simulink model "TVModel_Simulation_21"  (R2021b)
settings: Solver=FixedStepDiscrete  StartTime=0.0  StopTime=250  FixedStep=0.02  MaxStep=0.01  RelTol=1e-3
undefined symbols (not defined in the file or in its folder): MB, TV, TV_OLD
libraries: simulink x22, simulink_extras x14, eeGeneralControl x13, slpidlib x8, fuzblock x4, controlLib x4, cstblocks x3, dspstat3 x2, eeSlidingModeController x1, sharedTrackingLibrary x1
(part 2 of 9)

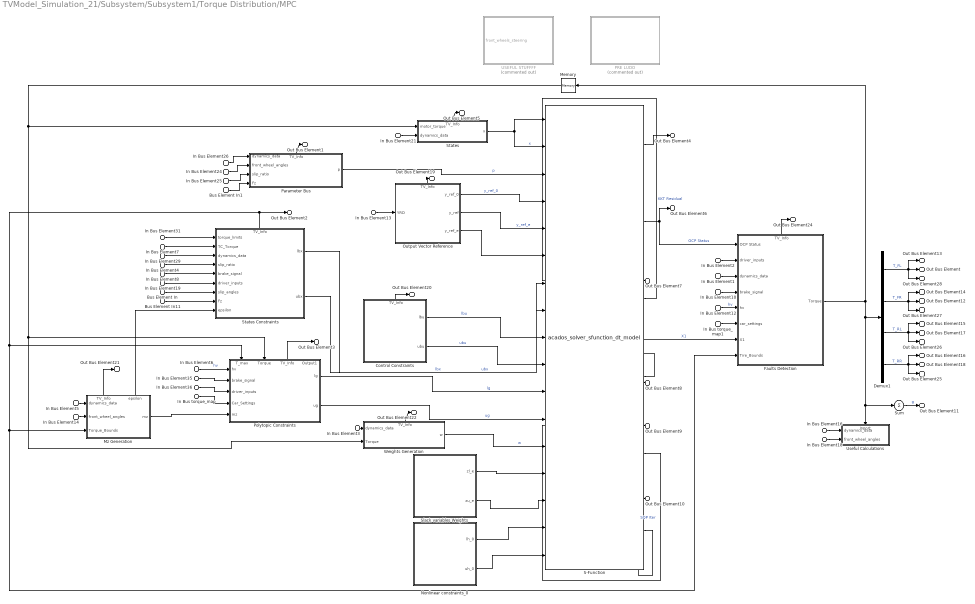
== system TVModel_Simulation_21/Subsystem/Subsystem1/Torque Distribution/MPC ==
  In Bus Element31 : Inport  PortName=torque_limits
  In Bus Element{1,3,5,16,21,26,29} (7 alike) : Inport  Port=2  PortName=dynamics_data
  In Bus Element13 : Inport  Port=3  PortName=yaw_rate_desired
  In Bus Element25 : Inport  Port=4  PortName=slip_ratio
  In Bus Element4 : Inport  Port=4  PortName=slip_ratio
  In Bus Element36 : Inport  Port=5  PortName=driver_inputs
  In Bus Element2 : Inport  Port=5  PortName=driver_inputs
  In Bus Element19 : Inport  Port=5  PortName=driver_inputs
  In Bus Element24 : Inport  Port=6  PortName=front_wheel_angles
  In Bus Element14 : Inport  Port=6  PortName=front_wheel_angles
  In Bus Element18 : Inport  Port=6  PortName=front_wheel_angles
  In Bus Element35 : Inport  Port=7  PortName=brake_signal
  In Bus Element8 : Inport  Port=7  PortName=brake_signal
  In Bus Element10 : Inport  Port=7  PortName=brake_signal
  In Bus Element7 : Inport  Port=8  PortName=TC_Torque
  In Bus torque_map : Inport  Port=9  PortName=Car_Setting
  In Bus torque_map1 : Inport  Port=9  PortName=Car_Setting
  In Bus Element6 : Inport  Port=10  PortName=hv
  In Bus Element12 : Inport  Port=10  PortName=hv
  Bus Element In : Inport  Port=11  PortName=slip_angles
  Bus Element In11 : Inport  Port=12  PortName=Fz
  Bus Element In1 : Inport  Port=12  PortName=Fz
  "     Output Vector Reference" : Subsystem
      settings: PortSchema="{\"entries\":[{\"content\":{\"sides\":[{\"content\":{\"connectorIds\":[\"In1\"]},\"type\":\"ConnectorPlacement.EquallySpacedRectSide\",\"uuid\":\"6eb43855-e5bb-45e2-8cd4-f053b217ea66\"},{\"content\":{\"connectorIds\":[\"Out1\",\"Out2\",\"Out3\"],\"side\":\"RIGHT\"},\"type\":\"ConnectorPlacement.EquallySpacedRectSide\",\"uuid\":\"38094b7e-63b6-42ff-9f99-20977d79efed\"},{\"content\":{\"connectorIds\":[\"Out4\"],\"side\":\"TOP\"},\"type\":\"ConnectorPlacement.EquallySpacedRectSide\",\"uuid\":\"9a3bf522-481b-4973-827b-befc16d2412c\"}]},\"type\":\"ConnectorPlacement.EquallySpacedConnector\",\"uuid\":\"c4e1068e-763d-4b01-8680-18fb7e18710b\"}],\"packageUris\":[\"http://schema.mathworks.com/mf0/Connector/R2020b\"],\"version\":\"1.0\"}"
  " PRE LUDO" : Subsystem  Commented=on
  " Parameter Bus " : Subsystem
      settings: PortSchema="{\"entries\":[{\"content\":{\"sides\":[{\"content\":{\"connectorIds\":[\"In1\",\"In2\",\"In3\",\"In4\"]},\"type\":\"ConnectorPlacement.EquallySpacedRectSide\",\"uuid\":\"a09562f1-0ace-4da8-b0ba-541877c845d4\"},{\"content\":{\"connectorIds\":[\"Out1\"],\"side\":\"RIGHT\"},\"type\":\"ConnectorPlacement.EquallySpacedRectSide\",\"uuid\":\"f2ac5cc5-a3cf-4f44-b665-78a7b5313457\"},{\"content\":{\"connectorIds\":[\"Out2\"],\"side\":\"TOP\"},\"type\":\"ConnectorPlacement.EquallySpacedRectSide\",\"uuid\":\"e9b1b537-1334-4243-8de4-5033dcf158b3\"}]},\"type\":\"ConnectorPlacement.EquallySpacedConnector\",\"uuid\":\"4a13e9e0-d022-4af6-9a72-5499c727e49d\"}],\"packageUris\":[\"http://schema.mathworks.com/mf0/Connector/R2020b\"],\"version\":\"1.0\"}"
  " States" : Subsystem
      settings: PortSchema="{\"entries\":[{\"content\":{\"sides\":[{\"content\":{\"connectorIds\":[\"In1\",\"In2\"]},\"type\":\"ConnectorPlacement.EquallySpacedRectSide\",\"uuid\":\"8d332d78-bc9f-4997-8663-87f4f2365fc7\"},{\"content\":{\"connectorIds\":[\"Out1\"],\"side\":\"RIGHT\"},\"type\":\"ConnectorPlacement.EquallySpacedRectSide\",\"uuid\":\"d5a2d93d-05d2-4fab-b578-55a6b40e1b7e\"},{\"content\":{\"connectorIds\":[\"Out2\"],\"side\":\"TOP\"},\"type\":\"ConnectorPlacement.EquallySpacedRectSide\",\"uuid\":\"85119e7a-0f7b-42a4-aa47-c419ac915ed1\"}]},\"type\":\"ConnectorPlacement.EquallySpacedConnector\",\"uuid\":\"bc00bdd8-907b-4556-9b65-7ae115265b2a\"}],\"packageUris\":[\"http://schema.mathworks.com/mf0/Connector/R2020b\"],\"version\":\"1.0\"}"
  Control Constraints : Subsystem
      settings: PortSchema="{\"entries\":[{\"content\":{\"sides\":[{\"content\":{\"connectorIds\":[]},\"type\":\"ConnectorPlacement.EquallySpacedRectSide\",\"uuid\":\"3047f7f6-6911-4b59-830a-220636e586ba\"},{\"content\":{\"connectorIds\":[\"Out1\",\"Out2\"],\"side\":\"RIGHT\"},\"type\":\"ConnectorPlacement.EquallySpacedRectSide\",\"uuid\":\"8d090d6d-9b64-48c1-acb0-b5c53a8577b5\"},{\"content\":{\"connectorIds\":[\"Out3\"],\"side\":\"TOP\"},\"type\":\"ConnectorPlacement.EquallySpacedRectSide\",\"uuid\":\"2db0e490-1b70-46d0-9c30-5c7bdf8b2a28\"}]},\"type\":\"ConnectorPlacement.EquallySpacedConnector\",\"uuid\":\"45990a81-75f2-4fb4-b041-5594cb9ed930\"}],\"packageUris\":[\"http://schema.mathworks.com/mf0/Connector/R2020b\"],\"version\":\"1.0\"}"
  Demux1 : Demux
  Faults Detection : Subsystem
      settings: PortSchema="{\"entries\":[{\"content\":{\"sides\":[{\"content\":{\"connectorIds\":[\"In1\",\"In2\",\"In3\",\"In4\",\"In5\",\"In6\",\"In7\",\"In8\"]},\"type\":\"ConnectorPlacement.EquallySpacedRectSide\",\"uuid\":\"334783ee-11f3-4144-8a14-28dc56086a4b\"},{\"content\":{\"connectorIds\":[\"Out1\"],\"side\":\"RIGHT\"},\"type\":\"ConnectorPlacement.EquallySpacedRectSide\",\"uuid\":\"49c8e620-bd09-4fee-a8d6-6c7a5f6563c1\"},{\"content\":{\"connectorIds\":[\"Out2\"],\"side\":\"TOP\"},\"type\":\"ConnectorPlacement.EquallySpacedRectSide\",\"uuid\":\"cef52ef8-f6f7-4321-a9c9-502de0ffc851\"}]},\"type\":\"ConnectorPlacement.EquallySpacedConnector\",\"uuid\":\"45428ca6-b9a3-4f64-8f7b-2072997d615d\"}],\"packageUris\":[\"http://schema.mathworks.com/mf0/Connector/R2020b\"],\"version\":\"1.0\"}"
  Memory : Memory  InheritSampleTime=on
  Mz Generation : Subsystem
      settings: PortSchema="{\"entries\":[{\"content\":{\"sides\":[{\"content\":{\"connectorIds\":[\"In1\",\"In2\",\"In3\"]},\"type\":\"ConnectorPlacement.EquallySpacedRectSide\",\"uuid\":\"12822615-03ad-45f6-8c43-45acae00b3c9\"},{\"content\":{\"connectorIds\":[\"Out1\"],\"side\":\"RIGHT\"},\"type\":\"ConnectorPlacement.EquallySpacedRectSide\",\"uuid\":\"651d1d31-9a4c-422b-aacb-e7edf3ade298\"},{\"content\":{\"connectorIds\":[\"Out2\",\"Out3\"],\"side\":\"TOP\"},\"type\":\"ConnectorPlacement.EquallySpacedRectSide\",\"uuid\":\"d0f71465-89ce-4a1f-947c-d935b63c1581\"}]},\"type\":\"ConnectorPlacement.EquallySpacedConnector\",\"uuid\":\"d07c68d3-c928-4ca4-a746-c386ba32e252\"}],\"packageUris\":[\"http://schema.mathworks.com/mf0/Connector/R2020b\"],\"version\":\"1.0\"}"
  Nonlinear constraints_0 : Subsystem
  Polytopic Constraints : Subsystem
      settings: PortSchema="{\"entries\":[{\"content\":{\"sides\":[{\"content\":{\"connectorIds\":[\"In1\",\"In2\",\"In3\",\"In4\",\"In5\"]},\"type\":\"ConnectorPlacement.EquallySpacedRectSide\",\"uuid\":\"e13c359e-3a3f-4544-8ddb-27eff3db9dcd\"},{\"content\":{\"connectorIds\":[\"Out1\",\"Out2\"],\"side\":\"RIGHT\"},\"type\":\"ConnectorPlacement.EquallySpacedRectSide\",\"uuid\":\"2a9e23e2-ef2f-461f-adc6-9f7488968d10\"},{\"content\":{\"connectorIds\":[\"In6\",\"In7\",\"Out3\",\"Out4\"],\"side\":\"TOP\"},\"type\":\"ConnectorPlacement.EquallySpacedRectSide\",\"uuid\":\"7b13a6d7-9b26-4287-8cf5-02c8da23c4d1\"}]},\"type\":\"ConnectorPlacement.EquallySpacedConnector\",\"uuid\":\"8c73910d-15b7-446d-b267-8db7451f6e4d\"}],\"packageUris\":[\"http://schema.mathworks.com/mf0/Connector/R2020b\"],\"version\":\"1.0\"}"
  S-Function : S-Function  FunctionName=acados_solver_sfunction_dt_model  SFunctionDeploymentMode=off  EnableBusSupport=off
  "Slack variables Weights " : Subsystem
  States Constraints : Subsystem
      settings: PortSchema="{\"entries\":[{\"content\":{\"sides\":[{\"content\":{\"connectorIds\":[\"In1\",\"In2\",\"In3\",\"In4\",\"In5\",\"In6\",\"In7\",\"In8\",\"In9\"]},\"type\":\"ConnectorPlacement.EquallySpacedRectSide\",\"uuid\":\"79113e7a-8644-4397-b81a-3f4227f55e88\"},{\"content\":{\"connectorIds\":[\"Out1\",\"Out2\"],\"side\":\"RIGHT\"},\"type\":\"ConnectorPlacement.EquallySpacedRectSide\",\"uuid\":\"08be16f7-b5e6-4d72-833b-a0e4a6b6f372\"},{\"content\":{\"connectorIds\":[\"Out3\"],\"side\":\"TOP\"},\"type\":\"ConnectorPlacement.EquallySpacedRectSide\",\"uuid\":\"49b46e5c-f00c-463e-b91e-3df34e18eb9d\"}]},\"type\":\"ConnectorPlacement.EquallySpacedConnector\",\"uuid\":\"b55b5f62-a08b-4632-a68f-4c31f9c7626d\"}],\"packageUris\":[\"http://schema.mathworks.com/mf0/Connector/R2020b\"],\"version\":\"1.0\"}"
  Sum : Sum  Inputs=+
  USEFUL STUFFFF : Subsystem  Commented=on
  Useful Calculations : Subsystem
      settings: PortSchema="{\"entries\":[{\"content\":{\"sides\":[{\"content\":{\"connectorIds\":[\"In1\",\"In2\"]},\"type\":\"ConnectorPlacement.EquallySpacedRectSide\",\"uuid\":\"a16c8cbd-7e59-4ceb-ae2f-8328deb35aba\"},{\"content\":{\"connectorIds\":[],\"side\":\"RIGHT\"},\"type\":\"ConnectorPlacement.EquallySpacedRectSide\",\"uuid\":\"ab644b37-73a3-4dcd-8f59-2df4491a3297\"},{\"content\":{\"connectorIds\":[\"In3\"],\"side\":\"TOP\"},\"type\":\"ConnectorPlacement.EquallySpacedRectSide\",\"uuid\":\"9843ece7-aa20-4f32-a700-0380b8b7d47e\"}]},\"type\":\"ConnectorPlacement.EquallySpacedConnector\",\"uuid\":\"e857cd10-f7b6-4e82-8686-4c399562f8ce\"}],\"packageUris\":[\"http://schema.mathworks.com/mf0/Connector/R2020b\"],\"version\":\"1.0\"}"
  Weights Generation : Subsystem
      settings: PortSchema="{\"entries\":[{\"content\":{\"sides\":[{\"content\":{\"connectorIds\":[\"In1\",\"In2\"]},\"type\":\"ConnectorPlacement.EquallySpacedRectSide\",\"uuid\":\"334783ee-11f3-4144-8a14-28dc56086a4b\"},{\"content\":{\"connectorIds\":[\"Out1\"],\"side\":\"RIGHT\"},\"type\":\"ConnectorPlacement.EquallySpacedRectSide\",\"uuid\":\"49c8e620-bd09-4fee-a8d6-6c7a5f6563c1\"},{\"content\":{\"connectorIds\":[\"Out2\"],\"side\":\"TOP\"},\"type\":\"ConnectorPlacement.EquallySpacedRectSide\",\"uuid\":\"cef52ef8-f6f7-4321-a9c9-502de0ffc851\"}]},\"type\":\"ConnectorPlacement.EquallySpacedConnector\",\"uuid\":\"45428ca6-b9a3-4f64-8f7b-2072997d615d\"}],\"packageUris\":[\"http://schema.mathworks.com/mf0/Connector/R2020b\"],\"version\":\"1.0\"}"
  Out Bus Element5 : Outport  PortName=TV_Info  Element=States
  Out Bus Element2 : Outport  PortName=TV_Info  Element=States_Constraints
  Out Bus Element3 : Outport  PortName=TV_Info  Element=Polytopic Constraints
  Out Bus Element4 : Outport  PortName=TV_Info  Element=control
  Out Bus Element6 : Outport  PortName=TV_Info  Element=Solver.OCP_status
  Out Bus Element7 : Outport  PortName=TV_Info  Element=Solver.KKT_Residual
  Out Bus Element8 : Outport  PortName=TV_Info  Element=Solver.X1
  Out Bus Element9 : Outport  PortName=TV_Info  Element=Solver.CPU_time
  Out Bus Element10 : Outport  PortName=TV_Info  Element=Solver.SQP_iter
  Out Bus Element16 : Outport  PortName=TV_Info  Element=Torque.t_rr
  Out Bus Element15 : Outport  PortName=TV_Info  Element=Torque.t_rl
  Out Bus Element14 : Outport  PortName=TV_Info  Element=Torque.t_fr
  Out Bus Element13 : Outport  PortName=TV_Info  Element=Torque.t_fl
  Out Bus Element11 : Outport  PortName=TV_Info  Element=Faults.g
  Out Bus Element1 : Outport  PortName=TV_Info  Element=Parameters
  Out Bus Element19 : Outport  PortName=TV_Info  Element=Vector_Reference
  Out Bus Element20 : Outport  PortName=TV_Info  Element=Control_Constraints
  Out Bus Element21 : Outport  PortName=TV_Info  Element=Mz_Saturation
  Out Bus Element22 : Outport  PortName=TV_Info  Element=Weights_Generation
  Out Bus Element24 : Outport  PortName=TV_Info  Element=Faults_Detection
  Out Bus Element : Outport  Port=2  PortName=TV  Element=FL
  Out Bus Element12 : Outport  Port=2  PortName=TV  Element=FR
  Out Bus Element17 : Outport  Port=2  PortName=TV  Element=RL
  Out Bus Element18 : Outport  Port=2  PortName=TV  Element=RR
  Out Bus Element25 : Outport  Port=3  PortName=TC_torque_out  Element=RR
  Out Bus Element26 : Outport  Port=3  PortName=TC_torque_out  Element=RL
  Out Bus Element27 : Outport  Port=3  PortName=TC_torque_out  Element=FR
  Out Bus Element28 : Outport  Port=3  PortName=TC_torque_out  Element=FL
  wires:
  Nonlinear constraints_0/2(uh_0) -> S-Function/17
  " States"/1(x) -> S-Function/1, S-Function/2  "x"
  In Bus Element21/1 -> " States"/2(dynamics_data)
  Mz Generation/3(epsilon) -> States Constraints/9(epsilon)
  In Bus Element18/1 -> Useful Calculations/2(front_wheel_angles)
  In Bus Element16/1 -> Useful Calculations/1(dynamics_data)
  Mz Generation/1(mz) -> Polytopic Constraints/5(mz)
  In Bus torque_map/1 -> Polytopic Constraints/4(Car_Settings)
  In Bus Element2/1 -> Faults Detection/2(driver_inputs)
  In Bus Element1/1 -> Faults Detection/3(dynamics_data)
  In Bus Element36/1 -> Polytopic Constraints/3(driver_inputs)
  In Bus Element35/1 -> Polytopic Constraints/2(brake_signal)
  In Bus Element24/1 -> " Parameter Bus "/2(front_wheel_angles)
  In Bus Element26/1 -> " Parameter Bus "/1(dynamics_data)
  In Bus Element25/1 -> " Parameter Bus "/3(slip_ratio)
  In Bus Element13/1 -> "     Output Vector Reference"/1(YRD)
  S-Function/5 -> Out Bus Element9/1
  S-Function/6 -> Out Bus Element10/1  "SQP Iter"
  S-Function/3 -> Out Bus Element7/1  "KKT Residual"
  S-Function/2 -> Faults Detection/1(OCP Status), Out Bus Element6/1  "OCP Status"
  Sum/1 -> Out Bus Element11/1  "g"
  Memory/1 -> " States"/1(motor_torque), Weights Generation/2(Torque), Polytopic Constraints/7(Torque)
  " States"/2(TV_Info) -> Out Bus Element5/1
  States Constraints/3(TV_Info) -> Faults Detection/8(Tire_Bounds), Mz Generation/3(Torque_Bounds), Polytopic Constraints/6(T_max), Out Bus Element2/1
  Polytopic Constraints/3(TV_Info) -> Out Bus Element3/1
  Demux1/1 -> Out Bus Element28/1, Out Bus Element/1, Out Bus Element13/1  "T_FL"
  Demux1/2 -> Out Bus Element27/1, Out Bus Element12/1, Out Bus Element14/1  "T_FR"
  Demux1/3 -> Out Bus Element26/1, Out Bus Element15/1, Out Bus Element17/1  "T_RL"
  Demux1/4 -> Out Bus Element25/1, Out Bus Element18/1, Out Bus Element16/1  "T_RR"
  In Bus Element3/1 -> Weights Generation/1(dynamics_data)
  S-Function/1 -> Out Bus Element4/1
  In Bus Element6/1 -> Polytopic Constraints/1(hv)  "hv"
  Faults Detection/1(Torque) -> Demux1/1, Sum/1, Useful Calculations/3(Inport), Memory/1
  " Parameter Bus "/2(TV_Info) -> Out Bus Element1/1
  "     Output Vector Reference"/4(TV_Info) -> Out Bus Element19/1
  Control Constraints/3(TV_Info) -> Out Bus Element20/1
  In Bus Element5/1 -> Mz Generation/1(dynamics_data)
  Mz Generation/2(TV_Info) -> Out Bus Element21/1
  Weights Generation/2(TV_Info) -> Out Bus Element22/1
  Faults Detection/2(TV_Info) -> Out Bus Element24/1
  In Bus Element14/1 -> Mz Generation/2(front_wheel_angles)
  In Bus Element12/1 -> Faults Detection/5(hv)  "hv"
  In Bus torque_map1/1 -> Faults Detection/6(car_settings)
  In Bus Element10/1 -> Faults Detection/4(brake_signal)
  Bus Element In11/1 -> States Constraints/8(Fz)
  Bus Element In/1 -> States Constraints/7(slip_angles)
  In Bus Element19/1 -> States Constraints/6(driver_inputs)
  In Bus Element8/1 -> States Constraints/5(brake_signal)
  In Bus Element4/1 -> States Constraints/4(slip_ratio)
  In Bus Element29/1 -> States Constraints/3(dynamics_data)
  In Bus Element7/1 -> States Constraints/2(TC_Torque)
  In Bus Element31/1 -> States Constraints/1(torque_limits)
  S-Function/4 -> Faults Detection/7(X1), Out Bus Element8/1  "X1"
  Bus Element In1/1 -> " Parameter Bus "/4(Fz)
  " Parameter Bus "/1(p) -> S-Function/3  "p"
  "     Output Vector Reference"/1(y_ref_0) -> S-Function/4  "y_ref_0"
  "     Output Vector Reference"/2(y_ref) -> S-Function/5  "y_ref_e"
  "     Output Vector Reference"/3(y_ref_e) -> S-Function/6
  States Constraints/1(lbx) -> S-Function/7  "lbx"
  States Constraints/2(ubx) -> S-Function/8  "ubx"
  Control Constraints/1(lbu) -> S-Function/9  "lbu"
  Control Constraints/2(ubu) -> S-Function/10  "ubu"
  Polytopic Constraints/1(lg) -> S-Function/11  "lg"
  Polytopic Constraints/2(ug) -> S-Function/12  "ug"
  Weights Generation/1(w) -> S-Function/13  "w"
  "Slack variables Weights "/1(zl_e) -> S-Function/14
  "Slack variables Weights "/2(zu_e) -> S-Function/15
  Nonlinear constraints_0/1(lh_0) -> S-Function/16

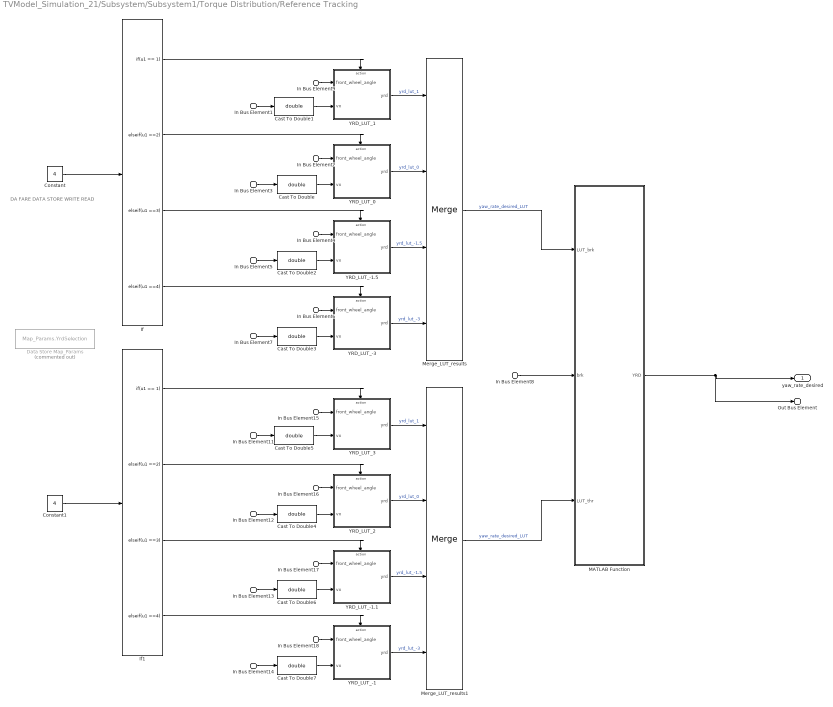
== system TVModel_Simulation_21/Subsystem/Subsystem1/Torque Distribution/Reference Tracking ==
  note: DA FARE DATA STORE WRITE READ
  In Bus Element{1,3,5,7,11..14} (8 alike) : Inport  PortName=dynamics_data  Element=vx
  In Bus Element{2,4,6,9,15..18} (8 alike) : Inport  Port=2  PortName=front_wheels_steering  Element=single_axis
  In Bus Element8 : Inport  Port=3  PortName=driver_inputs  Element=brake
  Cast To Double{,1..7} (8 alike) : DataTypeConversion  OutDataTypeStr=double
  Constant : Constant  Value=4
  Constant1 : Constant  Value=4
  Data Store Map_Params : DataStoreRead  Commented=on  DataStoreName=Map_Params  DataStoreElements=Map_Params.YrdSelection  IndexOptions=Index vector (dialog)  Indices=1  OutputSizes=1
  If : If  IfExpression=u1 == 1  ElseIfExpressions=u1 ==2,u1 ==3,u1 ==4  ShowElse=off
  If1 : If  IfExpression=u1 == 1  ElseIfExpressions=u1 ==2,u1 ==3,u1 ==4  ShowElse=off
  MATLAB Function : MATLAB Function  TreatAsAtomicUnit=on  SystemSampleTime=TV.MPC.T/TV.MPC.N
  Merge_LUT_results : Merge  Inputs=4
  Merge_LUT_results1 : Merge  Inputs=4
  YRD_LUT_-1 : Subsystem  TreatAsAtomicUnit=on
      mask Display: image('Mask_Icon\LUT.png'); % Use "Edit Image" on toolstrip to change.
  YRD_LUT_-1.1 : Subsystem  TreatAsAtomicUnit=on
      mask Display: image('Mask_Icon\LUT.png'); % Use "Edit Image" on toolstrip to change.
  YRD_LUT_-1.5 : Subsystem  TreatAsAtomicUnit=on
      mask Display: image('Mask_Icon\LUT.png'); % Use "Edit Image" on toolstrip to change.
  YRD_LUT_-3 : Subsystem  TreatAsAtomicUnit=on
      mask Display: image('Mask_Icon\LUT.png'); % Use "Edit Image" on toolstrip to change.
  YRD_LUT_0 : Subsystem  TreatAsAtomicUnit=on
      mask Display: image('Mask_Icon\LUT.png'); % Use "Edit Image" on toolstrip to change.
  YRD_LUT_1 : Subsystem  TreatAsAtomicUnit=on
      mask Display: image('Mask_Icon\LUT.png'); % Use "Edit Image" on toolstrip to change.
  YRD_LUT_2 : Subsystem  TreatAsAtomicUnit=on
      mask Display: image('Mask_Icon\LUT.png'); % Use "Edit Image" on toolstrip to change.
  YRD_LUT_3 : Subsystem  TreatAsAtomicUnit=on
      mask Display: image('Mask_Icon\LUT.png'); % Use "Edit Image" on toolstrip to change.
  yaw_rate_desired : Outport
  Out Bus Element : Outport  Port=2  PortName=TV_Info  Element=yaw_rate_desired
  wires:
  MATLAB Function/1(YRD) -> yaw_rate_desired/1, Out Bus Element/1
  In Bus Element8/1 -> MATLAB Function/2(brk)
  Constant1/1 -> If1/1
  Constant/1 -> If/1
  Merge_LUT_results/1 -> MATLAB Function/1(LUT_brk)  "yaw_rate_desired_LUT"
  Merge_LUT_results1/1 -> MATLAB Function/3(LUT_thr)  "yaw_rate_desired_LUT"
  In Bus Element15/1 -> YRD_LUT_3/1(front_wheel_angle)
  In Bus Element11/1 -> Cast To Double5/1
  In Bus Element16/1 -> YRD_LUT_2/1(front_wheel_angle)
  In Bus Element12/1 -> Cast To Double4/1
  In Bus Element17/1 -> YRD_LUT_-1.1/1(front_wheel_angle)
  In Bus Element13/1 -> Cast To Double6/1
  In Bus Element18/1 -> YRD_LUT_-1/1(front_wheel_angle)
  In Bus Element14/1 -> Cast To Double7/1
  If1/1 -> YRD_LUT_3/Action
  If1/2 -> YRD_LUT_2/Action
  If1/3 -> YRD_LUT_-1.1/Action
  If1/4 -> YRD_LUT_-1/Action
  YRD_LUT_-1/1(yrd) -> Merge_LUT_results1/4  "yrd_lut_-3"
  YRD_LUT_-1.1/1(yrd) -> Merge_LUT_results1/3  "yrd_lut_-1.5"
  YRD_LUT_3/1(yrd) -> Merge_LUT_results1/1  "yrd_lut_1"
  YRD_LUT_2/1(yrd) -> Merge_LUT_results1/2  "yrd_lut_0"
  Cast To Double4/1 -> YRD_LUT_2/2(vx)
  Cast To Double5/1 -> YRD_LUT_3/2(vx)
  Cast To Double6/1 -> YRD_LUT_-1.1/2(vx)
  Cast To Double7/1 -> YRD_LUT_-1/2(vx)
  Cast To Double3/1 -> YRD_LUT_-3/2(vx)
  Cast To Double2/1 -> YRD_LUT_-1.5/2(vx)
  Cast To Double1/1 -> YRD_LUT_1/2(vx)
  Cast To Double/1 -> YRD_LUT_0/2(vx)
  YRD_LUT_0/1(yrd) -> Merge_LUT_results/2  "yrd_lut_0"
  YRD_LUT_1/1(yrd) -> Merge_LUT_results/1  "yrd_lut_1"
  YRD_LUT_-1.5/1(yrd) -> Merge_LUT_results/3  "yrd_lut_-1.5"
  YRD_LUT_-3/1(yrd) -> Merge_LUT_results/4  "yrd_lut_-3"
  If/4 -> YRD_LUT_-3/Action
  If/3 -> YRD_LUT_-1.5/Action
  If/2 -> YRD_LUT_0/Action
  If/1 -> YRD_LUT_1/Action
  In Bus Element7/1 -> Cast To Double3/1
  In Bus Element6/1 -> YRD_LUT_-3/1(front_wheel_angle)
  In Bus Element5/1 -> Cast To Double2/1
  In Bus Element4/1 -> YRD_LUT_-1.5/1(front_wheel_angle)
  In Bus Element3/1 -> Cast To Double/1
  In Bus Element2/1 -> YRD_LUT_0/1(front_wheel_angle)
  In Bus Element1/1 -> Cast To Double1/1
  In Bus Element9/1 -> YRD_LUT_1/1(front_wheel_angle)

== system TVModel_Simulation_21/Subsystem/Subsystem1/Torque Limits/Torque Limits Positive ==
  In Bus torque_map1 : Inport  PortName=car_settings  Element=torque_map
  In Bus Element : Inport  Port=2  PortName=hv  Element=display_overload_motor
  In Bus Element1 : Inport  Port=2  PortName=hv  Element=display_overload_inverter
  In Bus Element6 : Inport  Port=3  PortName=dynamics_data  Element=omega_wheels
  Cast_{0..4} (5 alike) : DataTypeConversion
  Constant{,1..3} (4 alike) : Constant  Value=TV.LV.TORQUE.T_nominal_motor/1000*2200
  Constant4 : Constant  Value=0
  Constant5 : Constant  Value=0
  Constant6 : Constant  Value=0
  Constant7 : Constant  Value=540
  Max_Torque_Overload_Inverter_LUT : Lookup_n-D  NumberOfTableDimensions=1  BreakpointsForDimension1=[0 TV.LV.AMK.ID32999 1000]  Table=[TV.LV.AMK.ID82*TV.LV.AMK.ID32771/100 TV.LV.AMK.ID82*TV.LV.AMK.ID32771/100 0]  InternalRulePriority=Speed  RndMeth=Simplest  InputSameDT=on
  Max_Torque_Overload_Motor_LUT : Lookup_n-D  NumberOfTableDimensions=1  BreakpointsForDimension1=[0 TV.LV.AMK.ID114 1000]  Table=[TV.LV.AMK.ID82*TV.LV.AMK.ID32771/100 TV.LV.AMK.ID82*TV.LV.AMK.ID32771/100 0]  InternalRulePriority=Speed  RndMeth=Simplest  InputSameDT=on
  Max_Torque_Temperature_External_LUT : Lookup_n-D  NumberOfTableDimensions=1  BreakpointsForDimension1=[0 TV.LV.AMK.ID32798_11 TV.LV.AMK.ID32798_12]  Table=[TV.LV.AMK.ID82*TV.LV.AMK.ID32771/100 TV.LV.AMK.ID82*TV.LV.AMK.ID32771/100 0]  InternalRulePriority=Speed  RndMeth=Simplest  InputSameDT=on
  Max_Torque_Temperature_IGBT_LUT : Lookup_n-D  NumberOfTableDimensions=1  BreakpointsForDimension1=[0 TV.LV.AMK.ID32798_8 TV.LV.AMK.ID32798_9]  Table=[TV.LV.AMK.ID82*TV.LV.AMK.ID32771/100 TV.LV.AMK.ID82*TV.LV.AMK.ID32771/100 0]  InternalRulePriority=Speed  RndMeth=Simplest  InputSameDT=on
  Max_Torque_Temperature_Internal_LUT : Lookup_n-D  NumberOfTableDimensions=1  BreakpointsForDimension1=[0 TV.LV.AMK.ID32798_5 TV.LV.AMK.ID32798_6]  Table=[TV.LV.AMK.ID82*TV.LV.AMK.ID32771/100 TV.LV.AMK.ID82*TV.LV.AMK.ID32771/100 0]  InternalRulePriority=Speed  RndMeth=Simplest  InputSameDT=on
  Min : MinMax  Inputs=7
  Mux : Mux
  Saturation_Positive : Saturate  UpperLimit=+inf  LowerLimit=0
  Torque_Curve : Subsystem
  t_limit_positive : Outport
  wires:
  In Bus Element1/1 -> Cast_1/1  "display_overload_inverter"
  In Bus Element/1 -> Cast_0/1  "display_overload_motor"
  In Bus Element6/1 -> Torque_Curve/1(omega_wheels)  "omega_wheels"
  Max_Torque_Overload_Motor_LUT/1 -> Min/1  "max_torque_overload_motor"
  Max_Torque_Overload_Inverter_LUT/1 -> Min/2  "max_torque_overload_inverter_LUT"
  Max_Torque_Temperature_Internal_LUT/1 -> Min/3  "max_torque_temperature_internal"
  Max_Torque_Temperature_IGBT_LUT/1 -> Min/4  "max_torque_temperature_IGBT_LUT"
  In Bus torque_map1/1 -> Torque_Curve/3(torque_map)  "torque_map"
  Cast_0/1 -> Max_Torque_Overload_Motor_LUT/1
  Cast_1/1 -> Max_Torque_Overload_Inverter_LUT/1
  Cast_2/1 -> Max_Torque_Temperature_Internal_LUT/1
  Cast_3/1 -> Max_Torque_Temperature_IGBT_LUT/1
  Cast_4/1 -> Max_Torque_Temperature_External_LUT/1
  Min/1 -> Saturation_Positive/1  "t_limit"
  Max_Torque_Temperature_External_LUT/1 -> Min/5  "max_torque_temperature_external_LUT"
  Saturation_Positive/1 -> t_limit_positive/1  "t_limit_positive"
  Torque_Curve/1(max_torque_available) -> Min/6  "max_torque_available"
  Mux/1 -> Min/7
  Constant/1 -> Mux/1
  Constant1/1 -> Mux/2
  Constant2/1 -> Mux/3
  Constant3/1 -> Mux/4
  Constant4/1 -> Cast_3/1
  Constant5/1 -> Cast_4/1
  Constant6/1 -> Cast_2/1
  Constant7/1 -> Torque_Curve/2(voltage [ID380])

== system TVModel_Simulation_21/Subsystem/Subsystem1/Torque Limits/Torque Limits Regen ==
  note: cooling.tplate
  In Bus torque_map1 : Inport  PortName=car_settings  Element=torque_map
  In Bus Element : Inport  Port=2  PortName=hv  Element=display_overload_motor
  In Bus Element1 : Inport  Port=2  PortName=hv  Element=display_overload_inverter
  In Bus Element6 : Inport  Port=3  PortName=dynamics_data  Element=omega_wheels
  Cast_{0..4} (5 alike) : DataTypeConversion
  Constant{,1..3} (4 alike) : Constant  Value=21
  Constant4 : Constant  Value=0
  Constant5 : Constant  Value=0
  Constant6 : Constant  Value=0
  Constant7 : Constant  Value=540
  Display Overload Inverter LUT : Lookup_n-D  NumberOfTableDimensions=1  BreakpointsForDimension1=[0 TV.LV.AMK.ID32999 1000]  Table=[TV.LV.AMK.ID82*TV.LV.AMK.ID32771/100 TV.LV.AMK.ID82*TV.LV.AMK.ID32771/100 0]  InternalRulePriority=Speed  RndMeth=Simplest  InputSameDT=on
  Display Overload Motor LUT : Lookup_n-D  NumberOfTableDimensions=1  BreakpointsForDimension1=[0 TV.LV.AMK.ID114 1000]  Table=[TV.LV.AMK.ID82*TV.LV.AMK.ID32771/100 TV.LV.AMK.ID82*TV.LV.AMK.ID32771/100 0]  InternalRulePriority=Speed  RndMeth=Simplest  InputSameDT=on
  Min1 : MinMax  Inputs=7
  Mux : Mux
  Saturation_Positive : Saturate  UpperLimit=+inf  LowerLimit=0
  Temperature External LUT : Lookup_n-D  NumberOfTableDimensions=1  BreakpointsForDimension1=[0 TV.LV.AMK.ID32798_11 TV.LV.AMK.ID32798_12]  Table=[TV.LV.AMK.ID82*TV.LV.AMK.ID32771/100 TV.LV.AMK.ID82*TV.LV.AMK.ID32771/100 0]  InternalRulePriority=Speed  RndMeth=Simplest  InputSameDT=on
  Temperature IGBT LUT : Lookup_n-D  NumberOfTableDimensions=1  BreakpointsForDimension1=[0 TV.LV.AMK.ID32798_8 TV.LV.AMK.ID32798_9]  Table=[TV.LV.AMK.ID82*TV.LV.AMK.ID32771/100 TV.LV.AMK.ID82*TV.LV.AMK.ID32771/100 0]  InternalRulePriority=Speed  RndMeth=Simplest  InputSameDT=on
  Temperature Internal LUT : Lookup_n-D  NumberOfTableDimensions=1  BreakpointsForDimension1=[0 TV.LV.AMK.ID32798_5 TV.LV.AMK.ID32798_6]  Table=[TV.LV.AMK.ID82*TV.LV.AMK.ID32771/100 TV.LV.AMK.ID82*TV.LV.AMK.ID32771/100 0]  InternalRulePriority=Speed  RndMeth=Simplest  InputSameDT=on
  Torque_Curve : Subsystem
  t_limit_regen : Outport
  wires:
  Display Overload Inverter LUT/1 -> Min1/2  "max_torque_overload_inverter_LUT"
  In Bus torque_map1/1 -> Torque_Curve/3(torque_map)  "torque_map"
  Display Overload Motor LUT/1 -> Min1/1  "max_torque_overload_motor"
  Temperature External LUT/1 -> Min1/5  "max_torque_temperature_external_LUT"
  Cast_4/1 -> Temperature External LUT/1
  Min1/1 -> Saturation_Positive/1  "t_limit"
  Cast_0/1 -> Display Overload Motor LUT/1
  Temperature IGBT LUT/1 -> Min1/4  "max_torque_temperature_IGBT_LUT"
  Cast_3/1 -> Temperature IGBT LUT/1
  Constant5/1 -> Cast_4/1  "temperature_external"
  Cast_2/1 -> Temperature Internal LUT/1
  Cast_1/1 -> Display Overload Inverter LUT/1
  In Bus Element/1 -> Cast_0/1  "display_overload_motor"
  In Bus Element1/1 -> Cast_1/1  "display_overload_inverter"
  Temperature Internal LUT/1 -> Min1/3  "max_torque_temperature_internal"
  In Bus Element6/1 -> Torque_Curve/1(omega_wheels)  "omega_wheels"
  Saturation_Positive/1 -> t_limit_regen/1  "t_limit"
  Constant4/1 -> Cast_3/1  "temperature_IGBT"
  Torque_Curve/1(max_torque_available) -> Min1/6  "max_torque_available"
  Constant/1 -> Mux/1
  Constant2/1 -> Mux/3
  Mux/1 -> Min1/7
  Constant1/1 -> Mux/2
  Constant3/1 -> Mux/4
  Constant6/1 -> Cast_2/1
  Constant7/1 -> Torque_Curve/2(voltage [ID380])  "cooling.voltage"

== system TVModel_Simulation_21/Subsystem/Subsystem1/Slip Control/Load Transfer Calculation/Fz FL ==
  In Bus Element : Inport  PortName=dynamics_data  Element=ay
  In Bus Element1 : Inport  PortName=dynamics_data  Element=vx
  In Bus Element2 : Inport  PortName=dynamics_data  Element=ax
  Drag moment : Gain  Gain=0.5*TV.CAR.rho*TV.CAR.CdA*TV.CAR.hcop/TV.CAR.wb*0.5
  Lateral Load Transfer : Gain  Gain=TV.CAR.m/TV.CAR.tf*TV.CAR.hcog*0.5
  Lift Force : Gain  Gain=0.5*TV.CAR.rho*TV.CAR.ClA*(1-TV.CAR.xcop/TV.CAR.wb)*0.5
  Longitudinal Load Transfer : Gain  Gain=TV.CAR.m/TV.CAR.wb*TV.CAR.hcog*0.5
  Square1 : Math  Operator=square  SaturateOnIntegerOverflow=on
  Square2 : Math  Operator=square  SaturateOnIntegerOverflow=on
  Static Load Front : Constant  Value=TV.CAR.Fzf
  Subtract : Sum  Inputs=+++-+
  Unary Minus : UnaryMinus
  Unary Minus1 : UnaryMinus
  TV_Info : Outport
  wires:
  Lift Force/1 -> Subtract/3
  In Bus Element1/1 -> Square1/1, Square2/1
  Square2/1 -> Drag moment/1
  In Bus Element2/1 -> Unary Minus1/1
  Longitudinal Load Transfer/1 -> Subtract/5
  Lateral Load Transfer/1 -> Subtract/2
  Square1/1 -> Lift Force/1
  Static Load Front/1 -> Subtract/1
  Drag moment/1 -> Subtract/4
  Subtract/1 -> TV_Info/1
  In Bus Element/1 -> Unary Minus/1
  Unary Minus/1 -> Lateral Load Transfer/1
  Unary Minus1/1 -> Longitudinal Load Transfer/1

== system TVModel_Simulation_21/Subsystem/Subsystem1/Slip Control/Load Transfer Calculation/Fz FR ==
  In Bus Element : Inport  PortName=dynamics_data  Element=ay
  In Bus Element1 : Inport  PortName=dynamics_data  Element=vx
  In Bus Element2 : Inport  PortName=dynamics_data  Element=ax
  Drag moment : Gain  Gain=0.5*TV.CAR.rho*TV.CAR.CdA*TV.CAR.hcop/TV.CAR.wb*0.5
  Lateral Load Transfer : Gain  Gain=TV.CAR.m/TV.CAR.tf*TV.CAR.hcog*0.5
  Lift Force : Gain  Gain=0.5*TV.CAR.rho*TV.CAR.ClA*(1 - TV.CAR.xcop/TV.CAR.wb)*0.5
  Longitudinal Load Transfer : Gain  Gain=TV.CAR.m/TV.CAR.wb*TV.CAR.hcog*0.5
  Square1 : Math  Operator=square  SaturateOnIntegerOverflow=on
  Square2 : Math  Operator=square  SaturateOnIntegerOverflow=on
  Static Load Front : Constant  Value=TV.CAR.Fzf
  Subtract : Sum  Inputs=+-+-+
  Unary Minus : UnaryMinus
  Unary Minus1 : UnaryMinus
  TV_Info : Outport
  wires:
  Square2/1 -> Drag moment/1
  Lift Force/1 -> Subtract/3
  In Bus Element2/1 -> Unary Minus1/1
  Longitudinal Load Transfer/1 -> Subtract/5
  Lateral Load Transfer/1 -> Subtract/2
  Square1/1 -> Lift Force/1
  Static Load Front/1 -> Subtract/1
  In Bus Element1/1 -> Square2/1, Square1/1
  In Bus Element/1 -> Unary Minus/1
  Drag moment/1 -> Subtract/4
  Subtract/1 -> TV_Info/1
  Unary Minus/1 -> Lateral Load Transfer/1
  Unary Minus1/1 -> Longitudinal Load Transfer/1

== system TVModel_Simulation_21/Subsystem/Subsystem1/Slip Control/Load Transfer Calculation/Fz RL ==
  In Bus Element : Inport  PortName=dynamics_data  Element=ay
  In Bus Element1 : Inport  PortName=dynamics_data  Element=vx
  In Bus Element2 : Inport  PortName=dynamics_data  Element=ax
  Drag moment : Gain  Gain=0.5*TV.CAR.rho*TV.CAR.CdA*TV.CAR.hcop/TV.CAR.wb*0.5
  Lateral Load Transfer : Gain  Gain=TV.CAR.m/TV.CAR.tr*TV.CAR.hcog*0.5
  Lift Force : Gain  Gain=0.5*TV.CAR.rho*TV.CAR.ClA*(TV.CAR.xcop/TV.CAR.wb)*0.5
  Longitudinal Load Transfer : Gain  Gain=TV.CAR.m/TV.CAR.wb*TV.CAR.hcog*0.5
  Square1 : Math  Operator=square  SaturateOnIntegerOverflow=on
  Square2 : Math  Operator=square  SaturateOnIntegerOverflow=on
  Static Load Front : Constant  Value=TV.CAR.Fzr
  Subtract : Sum  Inputs=++++-
  Unary Minus : UnaryMinus
  Unary Minus1 : UnaryMinus
  TV_Info : Outport
  wires:
  In Bus Element1/1 -> Square1/1, Square2/1
  Square2/1 -> Drag moment/1
  Lift Force/1 -> Subtract/3
  In Bus Element2/1 -> Unary Minus1/1
  Longitudinal Load Transfer/1 -> Subtract/5
  Lateral Load Transfer/1 -> Subtract/2
  Square1/1 -> Lift Force/1
  Static Load Front/1 -> Subtract/1
  In Bus Element/1 -> Unary Minus/1
  Drag moment/1 -> Subtract/4
  Subtract/1 -> TV_Info/1
  Unary Minus/1 -> Lateral Load Transfer/1
  Unary Minus1/1 -> Longitudinal Load Transfer/1

== system TVModel_Simulation_21/Subsystem/Subsystem1/Slip Control/Load Transfer Calculation/Fz RR ==
  In Bus Element : Inport  PortName=dynamics_data  Element=ay
  In Bus Element1 : Inport  PortName=dynamics_data  Element=vx
  In Bus Element2 : Inport  PortName=dynamics_data  Element=ax
  Drag moment : Gain  Gain=0.5*TV.CAR.rho*TV.CAR.CdA*TV.CAR.hcop/TV.CAR.wb*0.5
  Lateral Load Transfer : Gain  Gain=TV.CAR.m/TV.CAR.tr*TV.CAR.hcog*0.5
  Lift Force : Gain  Gain=0.5*TV.CAR.rho*TV.CAR.ClA*(TV.CAR.xcop/TV.CAR.wb)*0.5
  Longitudinal Load Transfer : Gain  Gain=TV.CAR.m/TV.CAR.wb*TV.CAR.hcog*0.5
  Square1 : Math  Operator=square  SaturateOnIntegerOverflow=on
  Square2 : Math  Operator=square  SaturateOnIntegerOverflow=on
  Static Load Front : Constant  Value=TV.CAR.Fzr
  Subtract : Sum  Inputs=+-++-
  Unary Minus : UnaryMinus
  Unary Minus1 : UnaryMinus
  TV_Info : Outport
  wires:
  Square2/1 -> Drag moment/1
  Lift Force/1 -> Subtract/3
  In Bus Element2/1 -> Unary Minus1/1
  Longitudinal Load Transfer/1 -> Subtract/5
  Lateral Load Transfer/1 -> Subtract/2
  Square1/1 -> Lift Force/1
  Static Load Front/1 -> Subtract/1
  In Bus Element1/1 -> Square2/1, Square1/1
  In Bus Element/1 -> Unary Minus/1
  Drag moment/1 -> Subtract/4
  Subtract/1 -> TV_Info/1
  Unary Minus/1 -> Lateral Load Transfer/1
  Unary Minus1/1 -> Longitudinal Load Transfer/1

== system TVModel_Simulation_21/Subsystem/Subsystem1/Slip Control/Slip Angle Calculation/Slip Angle FL ==
  In Bus Element : Inport  PortName=dynamics_data  Element=vy
  In Bus Element1 : Inport  PortName=dynamics_data  Element=vx
  In Bus Element2 : Inport  PortName=dynamics_data  Element=yaw_rate
  In Bus Element3 : Inport  PortName=dynamics_data  Element=yaw_rate
  In Bus Element10 : Inport  Port=2  PortName=front_wheels_steering  Element=different_axis
  Atan : Trigonometry  Operator=atan2
  Gain : Gain  Gain=TV.CAR.a
  Gain1 : Gain  Gain=TV.CAR.tf/2
  Selector : Selector  InputPortWidth=2  IndexOptions=Index vector (dialog)  Indices=[1]  OutputSizes=1
  Subtract : Sum  Inputs=+-
  Subtract1 : Sum
  Subtract2 : Sum  Inputs=+-
  alpha_fl : Outport
  wires:
  In Bus Element10/1 -> Selector/1
  In Bus Element/1 -> Subtract1/1
  Atan/1 -> Subtract2/1
  Subtract1/1 -> Atan/1
  Subtract2/1 -> alpha_fl/1
  In Bus Element2/1 -> Gain/1
  Gain1/1 -> Subtract/2
  In Bus Element3/1 -> Gain1/1
  Gain/1 -> Subtract1/2
  Subtract/1 -> Atan/2
  In Bus Element1/1 -> Subtract/1
  Selector/1 -> Subtract2/2

== system TVModel_Simulation_21/Subsystem/Subsystem1/Slip Control/Slip Angle Calculation/Slip Angle FR ==
  In Bus Element : Inport  PortName=dynamics_data  Element=vy
  In Bus Element1 : Inport  PortName=dynamics_data  Element=vx
  In Bus Element2 : Inport  PortName=dynamics_data  Element=yaw_rate
  In Bus Element3 : Inport  PortName=dynamics_data  Element=yaw_rate
  In Bus Element12 : Inport  Port=2  PortName=front_wheel_angles  Element=different_axis
  Atan : Trigonometry  Operator=atan2
  Gain : Gain  Gain=TV.CAR.a
  Gain1 : Gain  Gain=TV.CAR.tf/2
  Selector : Selector  InputPortWidth=2  IndexOptions=Index vector (dialog)  Indices=[2]  OutputSizes=1
  Subtract : Sum
  Subtract1 : Sum
  Subtract2 : Sum  Inputs=+-
  alpha_fr : Outport
  wires:
  In Bus Element12/1 -> Selector/1
  In Bus Element3/1 -> Gain1/1
  In Bus Element1/1 -> Subtract/1
  In Bus Element2/1 -> Gain/1
  In Bus Element/1 -> Subtract1/1
  Atan/1 -> Subtract2/1
  Subtract1/1 -> Atan/1
  Subtract2/1 -> alpha_fr/1
  Gain1/1 -> Subtract/2
  Selector/1 -> Subtract2/2
  Gain/1 -> Subtract1/2
  Subtract/1 -> Atan/2

== system TVModel_Simulation_21/Subsystem/Subsystem1/Slip Control/Slip Angle Calculation/Slip Angle RL ==
  In Bus Element : Inport  PortName=dynamics_data  Element=vy
  In Bus Element1 : Inport  PortName=dynamics_data  Element=vx
  In Bus Element2 : Inport  PortName=dynamics_data  Element=yaw_rate
  In Bus Element3 : Inport  PortName=dynamics_data  Element=yaw_rate
  Atan : Trigonometry  Operator=atan2
  Gain : Gain  Gain=TV.CAR.b
  Gain1 : Gain  Gain=TV.CAR.tr/2
  Subtract : Sum  Inputs=+-
  Subtract1 : Sum  Inputs=+-
  alpha_rl : Outport
  wires:
  In Bus Element2/1 -> Gain/1
  In Bus Element/1 -> Subtract1/1
  In Bus Element3/1 -> Gain1/1
  In Bus Element1/1 -> Subtract/1
  Subtract1/1 -> Atan/1
  Atan/1 -> alpha_rl/1
  Gain1/1 -> Subtract/2
  Gain/1 -> Subtract1/2
  Subtract/1 -> Atan/2

== system TVModel_Simulation_21/Subsystem/Subsystem1/Slip Control/Slip Angle Calculation/Slip Angle RR ==
  In Bus Element : Inport  PortName=dynamics_data  Element=vy
  In Bus Element1 : Inport  PortName=dynamics_data  Element=vx
  In Bus Element2 : Inport  PortName=dynamics_data  Element=yaw_rate
  In Bus Element4 : Inport  PortName=dynamics_data  Element=yaw_rate
  Atan : Trigonometry  Operator=atan2
  Gain : Gain  Gain=TV.CAR.b
  Gain1 : Gain  Gain=TV.CAR.tr/2
  Subtract : Sum
  Subtract1 : Sum  Inputs=+-
  alpha_rr : Outport
  wires:
  In Bus Element4/1 -> Gain/1
  In Bus Element/1 -> Subtract1/1
  In Bus Element2/1 -> Gain1/1
  In Bus Element1/1 -> Subtract/1
  Subtract1/1 -> Atan/1
  Atan/1 -> alpha_rr/1
  Gain1/1 -> Subtract/2
  Gain/1 -> Subtract1/2
  Subtract/1 -> Atan/2

== system TVModel_Simulation_21/Subsystem/Subsystem1/Slip Control/Slip Ratios/FL SR ==
  In Bus Element : Inport  PortName=dynamics_data  Element=omega_wheels
  In Bus Element4 : Inport  PortName=dynamics_data  Element=vx
  In Bus Element2 : Inport  PortName=dynamics_data  Element=vx
  In Bus Element1 : Inport  PortName=dynamics_data  Element=vy
  In Bus Element6 : Inport  Port=2  PortName=front_wheels_steering  Element=different_axis
  Constant : Constant  Value=0
  Cos1 : Trigonometry  Operator=cos
  Cos2 : Trigonometry
  Divide4 : Product  Inputs=*/
  Divide5 : Product  Inputs=**
  Divide6 : Product  Inputs=**
  Gain3 : Gain  Gain=TV.CAR.rs
  Selector : Selector  InputPortWidth=4  IndexOptions=Index vector (dialog)  Indices=[1]  OutputSizes=1
  Selector1 : Selector  InputPortWidth=2  IndexOptions=Index vector (dialog)  Indices=[1]  OutputSizes=1
  Subtract3 : Sum  Inputs=+-
  Sum : Sum
  Switch : Switch  Criteria=u2 > Threshold  Threshold=0.5
  FL : Outport
  wires:
  In Bus Element/1 -> Selector/1  "fl"
  In Bus Element4/1 -> Switch/2
  Selector/1 -> Gain3/1
  Switch/1 -> FL/1
  Subtract3/1 -> Divide4/1
  Cos2/1 -> Divide6/1
  Sum/1 -> Divide4/2, Subtract3/2
  Cos1/1 -> Divide5/2
  Divide5/1 -> Sum/1
  Gain3/1 -> Subtract3/1
  Divide6/1 -> Sum/2
  In Bus Element2/1 -> Divide5/1
  In Bus Element1/1 -> Divide6/2
  Divide4/1 -> Switch/1  "FL"
  Constant/1 -> Switch/3
  Selector1/1 -> Cos1/1, Cos2/1
  In Bus Element6/1 -> Selector1/1

== system TVModel_Simulation_21/Subsystem/Subsystem1/Slip Control/Slip Ratios/FR SR ==
  In Bus Element : Inport  PortName=dynamics_data  Element=omega_wheels
  In Bus Element4 : Inport  PortName=dynamics_data  Element=vx
  In Bus Element2 : Inport  PortName=dynamics_data  Element=vx
  In Bus Element1 : Inport  PortName=dynamics_data  Element=vy
  In Bus Element6 : Inport  Port=2  PortName=front_wheels_steering  Element=different_axis
  Constant : Constant  Value=0
  Cos1 : Trigonometry  Operator=cos
  Cos2 : Trigonometry
  Divide4 : Product  Inputs=*/
  Divide5 : Product  Inputs=**
  Divide6 : Product  Inputs=**
  Gain3 : Gain  Gain=TV.CAR.rs
  Selector : Selector  InputPortWidth=4  IndexOptions=Index vector (dialog)  Indices=[2]  OutputSizes=1
  Selector1 : Selector  InputPortWidth=2  IndexOptions=Index vector (dialog)  Indices=[2]  OutputSizes=1
  Subtract3 : Sum  Inputs=+-
  Sum : Sum
  Switch : Switch  Criteria=u2 > Threshold  Threshold=0.5
  FR : Outport
  wires:
  Constant/1 -> Switch/3
  Divide4/1 -> Switch/1  "FL"
  In Bus Element1/1 -> Divide6/2
  In Bus Element2/1 -> Divide5/1
  Divide6/1 -> Sum/2
  Gain3/1 -> Subtract3/1
  Divide5/1 -> Sum/1
  Cos1/1 -> Divide5/2
  Sum/1 -> Subtract3/2, Divide4/2
  Cos2/1 -> Divide6/1
  Subtract3/1 -> Divide4/1
  Switch/1 -> FR/1
  In Bus Element/1 -> Selector/1  "fr"
  Selector/1 -> Gain3/1
  In Bus Element4/1 -> Switch/2
  Selector1/1 -> Cos2/1, Cos1/1
  In Bus Element6/1 -> Selector1/1

== system TVModel_Simulation_21/Subsystem/Subsystem1/Slip Control/Slip Ratios/RL RR  ==
  In Bus Element : Inport  PortName=dynamics_data  Element=omega_wheels
  In Bus Element1 : Inport  PortName=dynamics_data  Element=vx
  Constant : Constant  Value=0
  Divide : Product  Inputs=*/
  Gain : Gain  Gain=TV.CAR.rs
  Selector : Selector  InputPortWidth=4  IndexOptions=Index vector (dialog)  Indices=[4]  OutputSizes=1
  Subtract : Sum  Inputs=+-
  Switch : Switch  Criteria=u2 > Threshold  Threshold=0.5
  RR : Outport
  wires:
  Constant/1 -> Switch/3
  Divide/1 -> Switch/1  "RL"
  Switch/1 -> RR/1  "RR"
  Gain/1 -> Subtract/1
  Subtract/1 -> Divide/1
  In Bus Element1/1 -> Switch/2, Divide/2, Subtract/2
  In Bus Element/1 -> Selector/1  "rr"
  Selector/1 -> Gain/1

== system TVModel_Simulation_21/Subsystem/Subsystem1/Slip Control/Slip Ratios/RL SR ==
  In Bus Element : Inport  PortName=dynamics_data  Element=omega_wheels
  In Bus Element1 : Inport  PortName=dynamics_data  Element=vx
  Constant : Constant  Value=0
  Divide : Product  Inputs=*/
  Gain : Gain  Gain=TV.CAR.rs
  Selector : Selector  InputPortWidth=4  IndexOptions=Index vector (dialog)  Indices=[3]  OutputSizes=1
  Subtract : Sum  Inputs=+-
  Switch : Switch  Criteria=u2 > Threshold  Threshold=0.5
  RL : Outport
  wires:
  In Bus Element1/1 -> Subtract/2, Divide/2, Switch/2
  Subtract/1 -> Divide/1
  Gain/1 -> Subtract/1
  Switch/1 -> RL/1  "RL"
  Divide/1 -> Switch/1  "RL"
  Constant/1 -> Switch/3
  In Bus Element/1 -> Selector/1  "rl"
  Selector/1 -> Gain/1
